simulink model "TDE_based_BLF_Robot_Manipulation_20211106"  (R2021b)
settings: Solver=ode1  StartTime=0.0  StopTime=200  FixedStep=0.001  RelTol=1e-3  EnableMultiTasking=on
values from neighbouring files (symbols this model uses):
  g_bar_const = [ 100, 0.00 ... (first row only)    [Parameter_file.m]
  l_const = [ 0.8, 0.8 ... (first row only)    [Parameter_file.m]
  lowerBound = [ -0.2; -0.2 ]    [Parameter_file.m]
  upperBound = [ 0.25 ; 0.25 ]    [Parameter_file.m]
settings Model: Creator=59265  LastModifiedBy=59265

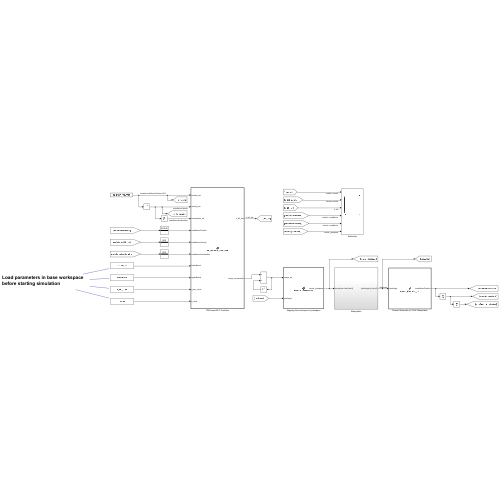
[thumbnail: Simulink's stored preview of the top-level diagram]
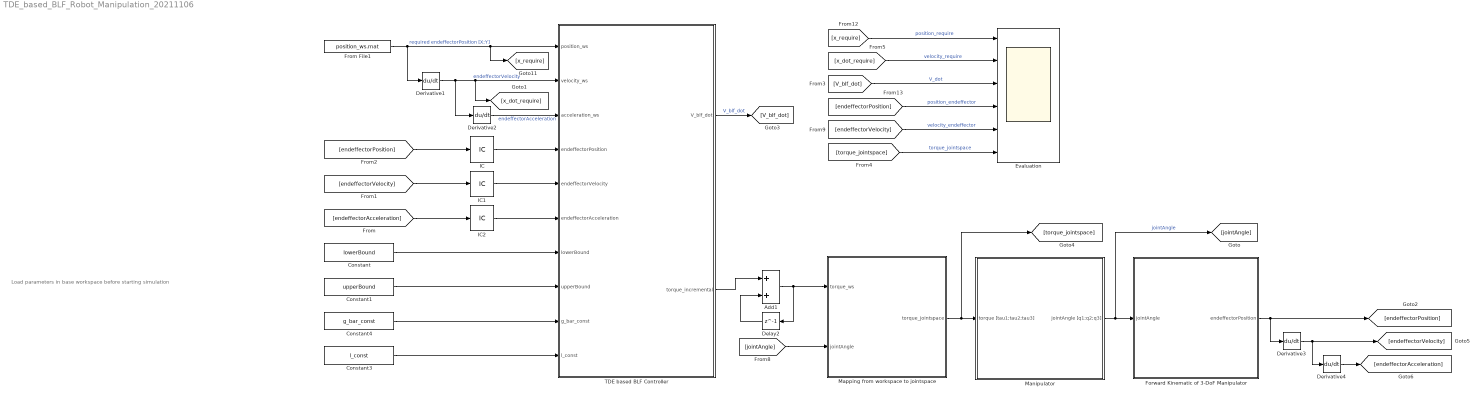
== system TDE_based_BLF_Robot_Manipulation_20211106 ==
  note: Load parameters in base workspace
      | before starting simulation
  Add1 : Sum
  Constant : Constant  Value=lowerBound
  Constant1 : Constant  Value=upperBound
  Constant3 : Constant  Value=l_const
  Constant4 : Constant  Value=g_bar_const
  Delay2 : Delay  DelayLength=1  InitialCondition=[0;0]
  Derivative{1..4} (4 alike) : Derivative
  Evaluation : Scope  NumInputPorts=6
  Forward Kinematic of 3-DoF Manipulator : MATLAB Function  TreatAsAtomicUnit=on
  From File1 : FromFile  FileName=position_ws.mat  SampleTime=0
  IC : InitialCondition  Value=[0.88;0]
  IC1 : InitialCondition  Value=[0;0]
  IC2 : InitialCondition  Value=[0;0]
  Manipulator : Subsystem
  Mapping from workspace to jointspace : MATLAB Function  TreatAsAtomicUnit=on
  TDE based BLF Controller : MATLAB Function  TreatAsAtomicUnit=on
  wires:
  Manipulator/1(jointAngle [q1;q2;q3]) -> Forward Kinematic of 3-DoF Manipulator/1(jointAngle), [jointAngle]  "jointAngle"
  TDE based BLF Controller/1(V_blf_dot) -> [V_blf_dot]  "V_blf_dot"
  Derivative2/1 -> TDE based BLF Controller/3(acceleration_ws)  "endeffectorAcceleration"
  Derivative1/1 -> Derivative2/1, [x_dot_require], TDE based BLF Controller/2(velocity_ws)  "endeffectorVelocity"
  Constant/1 -> TDE based BLF Controller/7(lowerBound)
  Constant1/1 -> TDE based BLF Controller/8(upperBound)
  Constant3/1 -> TDE based BLF Controller/10(l_const)
  Delay2/1 -> Add1/2
  TDE based BLF Controller/2(torque_incremental) -> Add1/1
  Mapping from workspace to jointspace/1(torque_jointspace) -> Manipulator/1(torque [tau1;tau2;tau3]), [torque_jointspace]
  From File1/1 -> Derivative1/1, [x_require], TDE based BLF Controller/1(position_ws)  "required endeffectorPosition [X;Y]"
  Constant4/1 -> TDE based BLF Controller/9(g_bar_const)
  [x_require] -> Evaluation/1  "position_require"
  [endeffectorPosition] -> Evaluation/4  "position_endeffector"
  [endeffectorVelocity] -> Evaluation/5  "velocity_endeffector"
  [x_dot_require] -> Evaluation/2  "velocity_require"
  [V_blf_dot] -> Evaluation/3  "V_dot"
  [torque_jointspace] -> Evaluation/6  "torque_jointspace"
  [jointAngle] -> Mapping from workspace to jointspace/2(jointAngle)
  Forward Kinematic of 3-DoF Manipulator/1(endeffectorPosition) -> Derivative3/1, [endeffectorPosition]
  Derivative3/1 -> Derivative4/1, [endeffectorVelocity]
  [endeffectorPosition] -> IC/1
  Derivative4/1 -> [endeffectorAcceleration]
  [endeffectorVelocity] -> IC1/1
  [endeffectorAcceleration] -> IC2/1
  IC/1 -> TDE based BLF Controller/4(endeffectorPosition)
  IC1/1 -> TDE based BLF Controller/5(endeffectorVelocity)
  IC2/1 -> TDE based BLF Controller/6(endeffectorAcceleration)
  Add1/1 -> Mapping from workspace to jointspace/1(torque_ws), Delay2/1

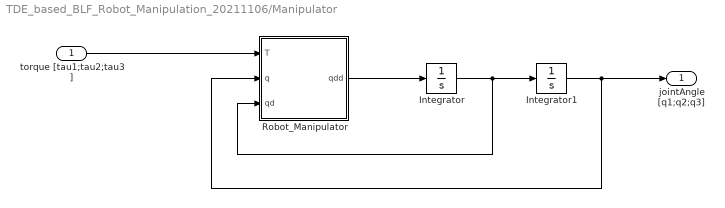
== system TDE_based_BLF_Robot_Manipulation_20211106/Manipulator ==
  torque [tau1;tau2;tau3] : Inport
  Integrator : Integrator  InitialCondition=[0;0;0]  ContinuousStateAttributes='velocity'
  Integrator1 : Integrator  InitialCondition=[0;0;0]  ContinuousStateAttributes='position'
  Robot_Manipulator : MATLAB Function  TreatAsAtomicUnit=on
  jointAngle [q1;q2;q3] : Outport  VectorParamsAs1DForOutWhenUnconnected=off
  wires:
  torque [tau1;tau2;tau3]/1 -> Robot_Manipulator/1(T)
  Robot_Manipulator/1(qdd) -> Integrator/1
  Integrator1/1 -> Robot_Manipulator/2(q), jointAngle [q1;q2;q3]/1
  Integrator/1 -> Robot_Manipulator/3(qd), Integrator1/1

== matlab function TDE_based_BLF_Robot_Manipulation_20211106/Forward Kinematic of 3-DoF Manipulator ==
  data: jointAngle input; endeffectorPosition output
function endeffectorPosition = forward_kinematic_calc(jointAngle)
% forward kinematic calculation for the 3-DoF Manipulator
% Transfer the given jointAngle to the position of endeffector in 2D workspace
%
%==========================================================================
% Input:             jointAngle          == angles of 3 DoF Manipulator with 3*1 Dimension
% Output:            endeffectorPosition == position of endeffector at 2D workspace [x;y] with 2*1 Dimension
% private variables: l1,l2,l3            == length of robot arm respectively
%==========================================================================

l1  = 0.30;
l2  = 0.24;
l3  = 0.34;
s1  = sin(jointAngle(1));
c1  = cos(jointAngle(1));
s12 = sin(jointAngle(1) + jointAngle(2));
c12 = cos(jointAngle(1) + jointAngle(2));
s123 = sin(jointAngle(1) + jointAngle(2) + jointAngle(3));
c123 = cos(jointAngle(1) + jointAngle(2) + jointAngle(3));

% forward kinematic of Robot arm
x = l1 * c1 + l2 * c12 + l3 * c123;
y = l1 * s1 + l2 * s12 + l3 * s123;

endeffectorPosition = [x;
                       y];

end

== matlab function TDE_based_BLF_Robot_Manipulation_20211106/TDE based BLF Controller ==
  data: position_ws input; velocity_ws input; acceleration_ws input; endeffectorPosition input; endeffectorVelocity input; V_blf_dot output; torque_incremental output; endeffectorAcceleration input; lowerBound input; upperBound input; g_bar_const input; l_const input
function [V_blf_dot, torque_incremental]  = blf_controller_calculation(position_ws, velocity_ws, acceleration_ws, ...
    endeffectorPosition, endeffectorVelocity, endeffectorAcceleration, lowerBound, upperBound, g_bar_const, l_const)
%% step 0: Announcement

% input:
%============================================================================
% position_ws               == Required Position of endeffector in X,Y planar workspace 2*N matrix
% velocity_ws               == Required Velocity of endeffector in X,Y planar workspace 2*N matrix
% acceleration_ws           == Required Acceleration of endeffector in X,Y planar workspace 2*N Matrix
% endeffectorPosition       == current position of endeffector in X,Y workspace == twice time integratin of x_2_dot
% endeffectorVelocity       == current velocity of endeffector in X,Y workspace == time integratin of x_2_dot
% endeffectorAcceleration   == current acceleration of endeffector in X,Y workspace == x_2_dot
% lowerBound                == lower limit of Position Error of endeffector with 2*1 Matrix for X,Y direction
% upperBound                == upper limit of Position Error of endeffector with 2*1 Matrix for X,Y direction
% l_const                   == constant values Matrix for calculation of LBF with 2*2 Dimension
% g_bar_const               == constant values Matirx with 2*2 Dimension
%============================================================================
%
% output:
%============================================================================
% V_blf_dot                 == time derivative of barrier Lyapnuov function, used for evaluation of stable system control
% torque_incremental        == required additional torque for the manipulator with 2*1 Dimension (in 2D workspace)
%============================================================================
%
% private variable:
%============================================================================
% P                         == coefficient of time derivative of BLF; V_1_dot = sum(e_1i*P(i)*e_1i_dot) 2*1 Vector
% A_Math_Term               == a math term that for calculation of alpha_dot which is equal to 
%                              P_dot(i)^(-1)*l_const_1i*positionError(1,i) + P(i)^(-1)*l_const_1i*positionError_dot(1,i)
% alpha                     == variable that make sure time derivative BLF function < 0, 2*1 Vector
% g_bar_const               == the core constant variable of this controller which indicates the performance of control loop
% l_const                   == the constant variable which related to the converge speed of lyapnouv function
%============================================================================

%% step 1: Translation joint angle into endeffector position and velocity 

x_1           = endeffectorPosition;                         % Position of endeffector in XY plane
x_2           = endeffectorVelocity;                         % Velocity of endeffector in XY plane

x_r_dot       = velocity_ws;                                 % requried time derivative of position = velocity_ws
x_r_dotdot    = acceleration_ws;                             % requried douple time derivative of position = acceleration_ws

%% step 2: dynamic system calculation using "Time Delay Estimation"

x_1_dot       = x_2;
x_2_dot       = endeffectorAcceleration;

%% step 3: barrier lyapunov function based for asymmetric contraints control

positionError = x_1 - position_ws;
positionError_dot = x_1_dot - x_r_dot; % e_1i_dot

% P_i with i = 1..2 is coefficient of time derivative of lyapnuov function first term
P_11 = (upperBound(1)^3 * lowerBound(1)^3 + upperBound(1)^2 * lowerBound(1)^2 * positionError(1,:)^2) /...
    ((upperBound(1) - positionError(1,:))^3 * (lowerBound(1) + positionError(1,:))^3);
P_21 = (upperBound(2)^3 * lowerBound(2)^3 + upperBound(2)^2 * lowerBound(2)^2 * positionError(2,:)^2) /...
    ((upperBound(2) - positionError(2,:))^3 * (lowerBound(2) + positionError(2,:))^3);
P = [P_11; P_21]; % 2*1 vector

P_dot_11 = (positionError_dot(1,:) * upperBound(1)^2 * lowerBound(1)^2 * (8*upperBound(1)*lowerBound(1)*positionError(1,:)...
    + 4 * positionError(1,:)^3 + (3 * upperBound(1) * lowerBound(1) + positionError(1,:)^2) * (lowerBound(1) - upperBound(1)) ))/...
    ((upperBound(1) - positionError(1))^4 * (lowerBound(1) + positionError(1))^4);
P_dot_21 = (positionError_dot(1,:) * upperBound(2)^2 * lowerBound(2)^2 * (8*upperBound(2)*lowerBound(2)*positionError(2,:)...
    + 4 * positionError(2,:)^3 + (3 * upperBound(2) * lowerBound(2) + positionError(2,:)^2) * (lowerBound(2) - upperBound(2)) ))/...
    ((upperBound(2) - positionError(2,:))^4 * (lowerBound(2) + positionError(2,:))^4);
P_dot = [P_dot_11; P_dot_21]; % 2*1 vector

% velocityError == x_2 - alpha, is a 2*1 vector
alpha_1 = velocity_ws(1,:) - P(1,1)^(-1) * l_const(1,1) * positionError(1,:);
alpha_2 = velocity_ws(2,:) - P(2,1)^(-1) * l_const(1,2) * positionError(2,:);
alpha = [alpha_1; alpha_2];

velocityError = x_2 - alpha;

%calculation of time derivative of alpha ---> alpha_dot
term_11 = - P_11^(-2) * P_dot_11 * l_const(1,1) * positionError(1) + P_11^(-1) * l_const(1,1) * positionError_dot(1);
term_21 = - P_21^(-2) * P_dot_21 * l_const(1,2) * positionError(2) + P_21^(-1) * l_const(1,2) * positionError_dot(2);
A_Math_Term = [term_11; term_21]; % 2*1 vector

alpha_dot = x_r_dotdot - A_Math_Term;

% torque incremental term calculation (delta u)
torque_incremental_1 = g_bar_const(1,1)^(-1) * alpha_dot(1) - g_bar_const(1,1)^(-1) * x_2_dot(1)...
    - l_const(2,1) * velocityError(1) - positionError(1) * P(1,1);
torque_incremental_2 = g_bar_const(2,2)^(-1) * alpha_dot(2) - g_bar_const(2,2)^(-1) * x_2_dot(2)...
    - l_const(2,2) * velocityError(2) - positionError(2) * P(2,1);
torque_incremental = [torque_incremental_1; torque_incremental_2]; % 2*1 Vector

% x_2_dot = x_2_0_dot + g_bar_const_pinv * torque_incremental;

% Conformation that the derivative of lyapnuov function should < 0  
V_blf_dot = -l_const(1,1) * positionError(1,:)^2 - l_const(2,1) * velocityError(1,:)...
    - l_const(1,2) * positionError(2,:)^2 - l_const(2,2) *velocityError(2,:);


end

== matlab function TDE_based_BLF_Robot_Manipulation_20211106/Mapping from workspace to jointspace ==
  data: torque_ws input; torque_jointspace output; jointAngle input
function torque_jointspace = mappingToJointspace(torque_ws, jointAngle)
% 3 DoF Manipulator
% Mapping the torque from workspace (2*1 Dimension) to jointspace (3*1 Dimension)
% Calculation of pseudo inverse of Jacobian Maxtrix (with J 3*2 Dimension)
J_pinv = pseudo_inverse_calc(jointAngle);

torque_jointspace = J_pinv * torque_ws;

== matlab function TDE_based_BLF_Robot_Manipulation_20211106/Manipulator/Robot_Manipulator ==
  data: T input; qdd output; q input; qd input
function qdd  = fcn(T,q,qd)
%#codegen

% cos and sine
c2 = cos(q(2));
c3 = cos(q(3));
c23 = cos(q(2)+q(3));
s2 = sin(q(2));
s3 = sin(q(3));
s23 = sin(q(2)+q(3));
% M-components
m11 = 1.0425+0.08094*c23+0.3484*c2+.0561*c3;
m12 = 0.4398+.04047*c23+.1742*c2+.0561*c3;
m13 = .1788+.04047*c23+.02809*c3;
m22 = .4398+.0519*c3;
m23 = .1788+.02809*c3;
m33 = .1788;
% Mass-Inertia matrix
M = [m11 m12 m13;
     m12 m22 m23;
     m13 m23 m33];
% N-components
n11 = -.1742*s2*qd(2)^2-0.04047*s23*qd(2)^2-.02809*s3*qd(3)^2-.04047*s23*qd(3)^2-0.3484*s2*qd(1)*qd(2)-.08094*s23*qd(1)*qd(2);
n12 = -0.05619*s3*qd(1)*qd(3)-.08094*s23*qd(1)*qd(3)-.05619*s3*qd(2)*qd(3)-.08094*s23*qd(2)*qd(3);
n2 = .1742*s2*qd(1)^2+.04047*s23*qd(1)^2-.02809*s3*qd(3)^2-0.0561*s3*qd(1)*qd(3)-0.05619*s3*qd(2)*qd(3);
n3 = 0.02809*s3*qd(1)^2+.02809*s3*qd(2)^2+.04047*s23*qd(1)^2+.05619*s3*qd(1)*qd(2);
% N matrix
N = [n11+n12;
     n2;
     n3];
% Friction coefficients
F = [2.6e-4 0 0;
     0 2.6e-4 0; 
     0 0 2.6e-4];

qdd=M\(T-N-F*qd);

end
